simulink model "OORT"  (Simulink 7.6)
settings: Solver=ode3  SolverMode=SingleTasking  StartTime=0.0  StopTime=1.2  FixedStep=2e-5  RelTol=1e-4  AbsTol=1e-6
undefined symbols (not defined in the file or in its folder): DAB, den, elements, num
libraries: powerlib x179, powerlib_extras x6
(part 2 of 4)

== system OORT/Off-Line Analysis/Line 3 ==
  Fault : Subsystem
  Fault Selector : Subsystem
  Line1 : powerlib/Elements/Distributed Parameters Line  DialogController=POWERSYS.PowerSysDialog  SystemSampleTime=-1  Phases=3  Frequency=ff  Resistance=rr  Inductance=ll  Capacitance=cc  Length=length*faultLocation  x1=[0 5.77041232459445e-009 110738.683831382 -249234.318095428;3.63428122191995e-005 5.73023176322571e-009 114142.922310078 -247693.751838263;7.26856244383991e-005 5.68897556743528e-009 117525.734769496 -246106.690441544;0.000109028436657599 5.64665148151452e-009 120886.486214459 -244473.431816059;0.000145371248876798 5.6032674502108e-009 124224.545790915 -242794.282544381;0.000181714061095998 5.55883161723614e-009 127539.286904351 -241069.557823317]  x2=[0 6.14623169531121e-009 110795.572141665 -250854.024226143;3.63428122191995e-005 6.10087361816961e-009 114221.996046724 -249312.526552019;7.26856244383991e-005 6.05437033260761e-009 117626.979089399 -247724.229874574;0.000109028436657599 6.00673056785934e-009 121009.882112826 -246089.432336475;0.000145371248876798 5.95796326648995e-009 124370.07010483 -244408.440809168;0.000181714061095998 5.90807758271694e-009 127706.912317124 -242681.570835272]  x3=[0 1.63289630452373e-011 297.327539148724 -989.32395322872;3.63428122191995e-005 1.63493812805236e-011 310.853854870665 -985.157566524455;7.26856244383991e-005 1.63667305374499e-011 324.321819531038 -980.806253724158;0.000109028436657599 1.63810075593491e-011 337.728905028542 -976.270831622334;0.000145371248876798 1.639220966625e-011 351.072594689637 -971.552151573052;0.000181714061095998 1.64003347553804e-011 364.350383740955 -966.651099330137]  x4=[0 -1.69443168699963e-012 498.560173361075 -967.719754733797;3.63428122191995e-005 -1.84264732192147e-012 511.771614093406 -960.798410267261;7.26856244383991e-005 -1.99051706945717e-012 524.886989049184 -953.696712215548;0.000109028436657599 -2.13801317265084e-012 537.903836312498 -946.415993654038;0.000145371248876798 -2.28510794468418e-012 550.819712462286 -938.957621262444;0.000181714061095998 -2.43177377407364e-012 563.632193030996 -931.32299506827]  x5=0.000181714061095998  Measurements=None
  Line2 : powerlib/Elements/Distributed Parameters Line  DialogController=POWERSYS.PowerSysDialog  SystemSampleTime=-1  Phases=3  Frequency=ff  Resistance=rr  Inductance=ll  Capacitance=cc  Length=length*(1-faultLocation)  x1=[0 6.14623169531121e-009 110795.572141665 -250854.024226143;3.63428122191995e-005 6.10087361816961e-009 114221.996046724 -249312.526552019;7.26856244383991e-005 6.05437033260761e-009 117626.979089399 -247724.229874574;0.000109028436657599 6.00673056785934e-009 121009.882112826 -246089.432336475;0.000145371248876798 5.95796326648995e-009 124370.07010483 -244408.440809168;0.000181714061095998 5.90807758271694e-009 127706.912317124 -242681.570835272]  x2=[0 6.09065079529943e-009 110951.105544523 -251348.844420414;3.63428122191995e-005 6.04474609507565e-009 114384.294130345 -249805.169420755;7.26856244383991e-005 5.99770672225242e-009 117796.011388453 -248214.602942697;0.000109028436657599 5.94954150669399e-009 121185.616897888 -246577.443554977;0.000145371248876798 5.90025948959903e-009 124552.474388336 -244893.998572387;0.000181714061095998 5.84986992180347e-009 127895.951859564 -243164.583998093]  x3=[0 1.03895542727053e-011 368.109218234945 -994.520254979836;3.63428122191995e-005 1.03400987350235e-011 381.70008253833 -989.383636970479;7.26856244383991e-005 1.02887022346403e-011 395.219297078756 -984.0612995801;0.000109028436657599 1.02353744193059e-011 408.664324134692 -978.554241876369;0.000145371248876798 1.01801252993019e-011 422.032639910506 -972.863497601215;0.000181714061095998 1.01229652455624e-011 435.321735010208 -966.990134976776]  x4=[0 6.77730234632808e-012 428.347420618646 -970.712392687894;3.63428122191995e-005 6.74770065951855e-012 441.606451848913 -964.752716375506;7.26856244383991e-005 6.71683234696046e-012 454.782588159728 -958.611944206436;0.000109028436657599 6.6847032030127e-012 467.873356229534 -952.291228878548;0.000145371248876798 6.65131925870764e-012 480.87629876143 -945.791756867236;0.000181714061095998 6.61668678061897e-012 493.788974944442 -939.1147482027]  x5=0.000181714061095998  Measurements=None
  Timer : powerlib_extras/Control  Blocks/Timer  DialogController=POWERSYS.PowerSysDialog  SystemSampleTime=-1  t=[0 faultTime]  e=[0 1 0 1 0 1]
  A1 : PMIOPort  Tag=PMCPort  Port=1  Side=Left
  B1 : PMIOPort  Tag=PMCPort  Port=2  Side=Left
  C1 : PMIOPort  Tag=PMCPort  Port=3  Side=Left
  A2 : PMIOPort  Tag=PMCPort  Port=4  Side=Right
  B2 : PMIOPort  Tag=PMCPort  Port=5  Side=Right
  C2 : PMIOPort  Tag=PMCPort  Port=6  Side=Right
  wires:
  Fault Selector/1(faultA) -> Fault/1(faultA)
  Fault Selector/2(faultB) -> Fault/2(faultB)
  Fault Selector/3(faultC) -> Fault/3(faultC)
  Fault Selector/4(faultG) -> Fault/4(faultG)
  Timer/1 -> Fault/5(Tfault)
  connections:
  Line1/RConn1 -- Line2/LConn1 -- Fault/LConn1
  Line1/RConn2 -- Line2/LConn2 -- Fault/LConn2
  Line2/LConn3 -- Line1/RConn3 -- Fault/LConn3
  A1/RConn1 -- Line1/LConn1
  B1/RConn1 -- Line1/LConn2
  C1/RConn1 -- Line1/LConn3
  Line2/RConn1 -- A2/RConn1
  Line2/RConn2 -- B2/RConn1
  Line2/RConn3 -- C2/RConn1

== system OORT/On-Line Analysis/CB-1 ==
  Trip : Inport
  BreakerA : powerlib/Elements/Breaker  DialogController=POWERSYS.PowerSysDialog  SystemSampleTime=-1  BreakerResistance=0.01  InitialState=1  SnubberResistance=1e6  SnubberCapacitance=inf  SwitchingTimes="[ 1/60  5/60 ]"  External=on  Measurements=None  MoreParameters=off  NoBreakLoop=off
  BreakerB : powerlib/Elements/Breaker  DialogController=POWERSYS.PowerSysDialog  SystemSampleTime=-1  BreakerResistance=0.01  InitialState=1  SnubberResistance=1e6  SnubberCapacitance=inf  SwitchingTimes="[ 1/60  5/60 ]"  External=on  Measurements=None  MoreParameters=off  NoBreakLoop=off
  BreakerC : powerlib/Elements/Breaker  DialogController=POWERSYS.PowerSysDialog  SystemSampleTime=-1  BreakerResistance=0.01  InitialState=1  SnubberResistance=1e6  SnubberCapacitance=inf  SwitchingTimes="[ 1/60  5/60 ]"  External=on  Measurements=None  MoreParameters=off  NoBreakLoop=off
  NOT : Logic  Operator=NOT  Inputs=1
  Series RLC Branch1 : powerlib/Elements/Series RLC Branch  DialogController=POWERSYS.PowerSysDialog  PhysicalDomain=powersysdomain  SubClassName=unknown  LeftPortType=p1  RightPortType=p1  LConnTagsString=__new0  RConnTagsString=__new0  BranchType=R  Resistance=1e6  Inductance=1.0  SetiL0=off  InitialCurrent=0  Capacitance=1.0  Setx0=off  InitialVoltage=0  Measurements=None
  Series RLC Branch2 : powerlib/Elements/Series RLC Branch  DialogController=POWERSYS.PowerSysDialog  PhysicalDomain=powersysdomain  SubClassName=unknown  LeftPortType=p1  RightPortType=p1  LConnTagsString=__new0  RConnTagsString=__new0  BranchType=R  Resistance=1e6  Inductance=1.0  SetiL0=off  InitialCurrent=0  Capacitance=1.0  Setx0=off  InitialVoltage=0  Measurements=None
  Series RLC Branch3 : powerlib/Elements/Series RLC Branch  DialogController=POWERSYS.PowerSysDialog  PhysicalDomain=powersysdomain  SubClassName=unknown  LeftPortType=p1  RightPortType=p1  LConnTagsString=__new0  RConnTagsString=__new0  BranchType=R  Resistance=1e6  Inductance=1.0  SetiL0=off  InitialCurrent=0  Capacitance=1.0  Setx0=off  InitialVoltage=0  Measurements=None
  Transport Delay : TransportDelay  DelayTime=t_op+0.001  BufferSize=10240
  A1 : PMIOPort  Tag=PMCPort  Port=1  Side=Left
  B1 : PMIOPort  Tag=PMCPort  Port=2  Side=Left
  C1 : PMIOPort  Tag=PMCPort  Port=3  Side=Left
  A2 : PMIOPort  Tag=PMCPort  Port=4  Side=Right
  B2 : PMIOPort  Tag=PMCPort  Port=5  Side=Right
  C2 : PMIOPort  Tag=PMCPort  Port=6  Side=Right
  wires:
  NOT/1 -> BreakerA/1, BreakerB/1, BreakerC/1
  Transport Delay/1 -> NOT/1
  Trip/1 -> Transport Delay/1
  connections:
  A2/RConn1 -- BreakerA/RConn1 -- Series RLC Branch1/RConn1
  B2/RConn1 -- BreakerB/RConn1 -- Series RLC Branch2/RConn1
  C2/RConn1 -- BreakerC/RConn1 -- Series RLC Branch3/RConn1
  A1/RConn1 -- BreakerA/LConn1 -- Series RLC Branch1/LConn1
  B1/RConn1 -- BreakerB/LConn1 -- Series RLC Branch2/LConn1
  C1/RConn1 -- BreakerC/LConn1 -- Series RLC Branch3/LConn1

== system OORT/On-Line Analysis/CB-2 ==
  Trip : Inport
  BreakerA : powerlib/Elements/Breaker  DialogController=POWERSYS.PowerSysDialog  SystemSampleTime=-1  BreakerResistance=0.01  InitialState=1  SnubberResistance=1e6  SnubberCapacitance=inf  SwitchingTimes="[ 1/60  5/60 ]"  External=on  Measurements=None  MoreParameters=off  NoBreakLoop=off
  BreakerB : powerlib/Elements/Breaker  DialogController=POWERSYS.PowerSysDialog  SystemSampleTime=-1  BreakerResistance=0.01  InitialState=1  SnubberResistance=1e6  SnubberCapacitance=inf  SwitchingTimes="[ 1/60  5/60 ]"  External=on  Measurements=None  MoreParameters=off  NoBreakLoop=off
  BreakerC : powerlib/Elements/Breaker  DialogController=POWERSYS.PowerSysDialog  SystemSampleTime=-1  BreakerResistance=0.01  InitialState=1  SnubberResistance=1e6  SnubberCapacitance=inf  SwitchingTimes="[ 1/60  5/60 ]"  External=on  Measurements=None  MoreParameters=off  NoBreakLoop=off
  NOT : Logic  Operator=NOT  Inputs=1
  Series RLC Branch1 : powerlib/Elements/Series RLC Branch  DialogController=POWERSYS.PowerSysDialog  PhysicalDomain=powersysdomain  SubClassName=unknown  LeftPortType=p1  RightPortType=p1  LConnTagsString=__new0  RConnTagsString=__new0  BranchType=R  Resistance=1e6  Inductance=1.0  SetiL0=off  InitialCurrent=0  Capacitance=1.0  Setx0=off  InitialVoltage=0  Measurements=None
  Series RLC Branch2 : powerlib/Elements/Series RLC Branch  DialogController=POWERSYS.PowerSysDialog  PhysicalDomain=powersysdomain  SubClassName=unknown  LeftPortType=p1  RightPortType=p1  LConnTagsString=__new0  RConnTagsString=__new0  BranchType=R  Resistance=1e6  Inductance=1.0  SetiL0=off  InitialCurrent=0  Capacitance=1.0  Setx0=off  InitialVoltage=0  Measurements=None
  Series RLC Branch3 : powerlib/Elements/Series RLC Branch  DialogController=POWERSYS.PowerSysDialog  PhysicalDomain=powersysdomain  SubClassName=unknown  LeftPortType=p1  RightPortType=p1  LConnTagsString=__new0  RConnTagsString=__new0  BranchType=R  Resistance=1e6  Inductance=1.0  SetiL0=off  InitialCurrent=0  Capacitance=1.0  Setx0=off  InitialVoltage=0  Measurements=None
  Transport Delay : TransportDelay  DelayTime=t_op+0.001  BufferSize=10240
  A1 : PMIOPort  Tag=PMCPort  Port=1  Side=Left
  B1 : PMIOPort  Tag=PMCPort  Port=2  Side=Left
  C1 : PMIOPort  Tag=PMCPort  Port=3  Side=Left
  A2 : PMIOPort  Tag=PMCPort  Port=4  Side=Right
  B2 : PMIOPort  Tag=PMCPort  Port=5  Side=Right
  C2 : PMIOPort  Tag=PMCPort  Port=6  Side=Right
  wires:
  Trip/1 -> Transport Delay/1
  Transport Delay/1 -> NOT/1
  NOT/1 -> BreakerC/1, BreakerB/1, BreakerA/1
  connections:
  Series RLC Branch3/LConn1 -- BreakerC/LConn1 -- C1/RConn1
  Series RLC Branch2/LConn1 -- BreakerB/LConn1 -- B1/RConn1
  Series RLC Branch1/LConn1 -- BreakerA/LConn1 -- A1/RConn1
  Series RLC Branch3/RConn1 -- BreakerC/RConn1 -- C2/RConn1
  Series RLC Branch2/RConn1 -- BreakerB/RConn1 -- B2/RConn1
  Series RLC Branch1/RConn1 -- BreakerA/RConn1 -- A2/RConn1

== system OORT/On-Line Analysis/CB-3 ==
  Trip : Inport
  BreakerA : powerlib/Elements/Breaker  DialogController=POWERSYS.PowerSysDialog  SystemSampleTime=-1  BreakerResistance=0.01  InitialState=1  SnubberResistance=1e6  SnubberCapacitance=inf  SwitchingTimes="[ 1/60  5/60 ]"  External=on  Measurements=None  MoreParameters=off  NoBreakLoop=off
  BreakerB : powerlib/Elements/Breaker  DialogController=POWERSYS.PowerSysDialog  SystemSampleTime=-1  BreakerResistance=0.01  InitialState=1  SnubberResistance=1e6  SnubberCapacitance=inf  SwitchingTimes="[ 1/60  5/60 ]"  External=on  Measurements=None  MoreParameters=off  NoBreakLoop=off
  BreakerC : powerlib/Elements/Breaker  DialogController=POWERSYS.PowerSysDialog  SystemSampleTime=-1  BreakerResistance=0.01  InitialState=1  SnubberResistance=1e6  SnubberCapacitance=inf  SwitchingTimes="[ 1/60  5/60 ]"  External=on  Measurements=None  MoreParameters=off  NoBreakLoop=off
  NOT : Logic  Operator=NOT  Inputs=1
  Series RLC Branch1 : powerlib/Elements/Series RLC Branch  DialogController=POWERSYS.PowerSysDialog  PhysicalDomain=powersysdomain  SubClassName=unknown  LeftPortType=p1  RightPortType=p1  LConnTagsString=__new0  RConnTagsString=__new0  BranchType=R  Resistance=1e6  Inductance=1.0  SetiL0=off  InitialCurrent=0  Capacitance=1.0  Setx0=off  InitialVoltage=0  Measurements=None
  Series RLC Branch2 : powerlib/Elements/Series RLC Branch  DialogController=POWERSYS.PowerSysDialog  PhysicalDomain=powersysdomain  SubClassName=unknown  LeftPortType=p1  RightPortType=p1  LConnTagsString=__new0  RConnTagsString=__new0  BranchType=R  Resistance=1e6  Inductance=1.0  SetiL0=off  InitialCurrent=0  Capacitance=1.0  Setx0=off  InitialVoltage=0  Measurements=None
  Series RLC Branch3 : powerlib/Elements/Series RLC Branch  DialogController=POWERSYS.PowerSysDialog  PhysicalDomain=powersysdomain  SubClassName=unknown  LeftPortType=p1  RightPortType=p1  LConnTagsString=__new0  RConnTagsString=__new0  BranchType=R  Resistance=1e6  Inductance=1.0  SetiL0=off  InitialCurrent=0  Capacitance=1.0  Setx0=off  InitialVoltage=0  Measurements=None
  Transport Delay : TransportDelay  DelayTime=t_op+0.001  BufferSize=10240
  A1 : PMIOPort  Tag=PMCPort  Port=1  Side=Left
  B1 : PMIOPort  Tag=PMCPort  Port=2  Side=Left
  C1 : PMIOPort  Tag=PMCPort  Port=3  Side=Left
  A2 : PMIOPort  Tag=PMCPort  Port=4  Side=Right
  B2 : PMIOPort  Tag=PMCPort  Port=5  Side=Right
  C2 : PMIOPort  Tag=PMCPort  Port=6  Side=Right
  wires:
  NOT/1 -> BreakerA/1, BreakerB/1, BreakerC/1
  Transport Delay/1 -> NOT/1
  Trip/1 -> Transport Delay/1
  connections:
  A2/RConn1 -- BreakerA/RConn1 -- Series RLC Branch1/RConn1
  B2/RConn1 -- BreakerB/RConn1 -- Series RLC Branch2/RConn1
  C2/RConn1 -- BreakerC/RConn1 -- Series RLC Branch3/RConn1
  A1/RConn1 -- BreakerA/LConn1 -- Series RLC Branch1/LConn1
  B1/RConn1 -- BreakerB/LConn1 -- Series RLC Branch2/LConn1
  C1/RConn1 -- BreakerC/LConn1 -- Series RLC Branch3/LConn1

== system OORT/On-Line Analysis/CT-1 ==
  CT-ratio : Gain  Gain=1/CT  SaturateOnIntegerOverflow=on  OutDataTypeStr=Inherit: Same as input  ParamDataTypeStr=Inherit: Same as input
  Ground : powerlib/Elements/Ground  DialogController=POWERSYS.PowerSysDialog  PhysicalDomain=powersysdomain  SubClassName=unknown  LeftPortType=p1  RightPortType=p1  LConnTagsString=a
  IA : powerlib/Measurements/Current Measurement  DialogController=POWERSYS.PowerSysDialog  SystemSampleTime=-1  PhasorSimulation=off  OutputType=Complex  PSBequivalent=0
  IB : powerlib/Measurements/Current Measurement  DialogController=POWERSYS.PowerSysDialog  SystemSampleTime=-1  PhasorSimulation=off  OutputType=Complex  PSBequivalent=0
  IC : powerlib/Measurements/Current Measurement  DialogController=POWERSYS.PowerSysDialog  SystemSampleTime=-1  PhasorSimulation=off  OutputType=Complex  PSBequivalent=0
  Mux : Mux  Inputs=3
  Mux1 : Mux  Inputs=3
  VA : powerlib/Measurements/Voltage Measurement  DialogController=POWERSYS.PowerSysDialog  SystemSampleTime=-1  PhasorSimulation=off  OutputType=Complex  PSBequivalent=0
  VB : powerlib/Measurements/Voltage Measurement  DialogController=POWERSYS.PowerSysDialog  SystemSampleTime=-1  PhasorSimulation=off  OutputType=Complex  PSBequivalent=0
  VC : powerlib/Measurements/Voltage Measurement  DialogController=POWERSYS.PowerSysDialog  SystemSampleTime=-1  PhasorSimulation=off  OutputType=Complex  PSBequivalent=0
  VT-ratio : Gain  Gain=1/VT  SaturateOnIntegerOverflow=on  OutDataTypeStr=Inherit: Same as input  ParamDataTypeStr=Inherit: Same as input
  A1 : PMIOPort  Tag=PMCPort  Port=1  Side=Left
  B1 : PMIOPort  Tag=PMCPort  Port=2  Side=Left
  C1 : PMIOPort  Tag=PMCPort  Port=3  Side=Left
  A2 : PMIOPort  Tag=PMCPort  Port=4  Side=Right
  B2 : PMIOPort  Tag=PMCPort  Port=5  Side=Right
  C2 : PMIOPort  Tag=PMCPort  Port=6  Side=Right
  Vabc : Outport  InitialOutput=0
  Iabc : Outport  Port=2  InitialOutput=0
  wires:
  VC/1 -> Mux1/3
  VB/1 -> Mux1/2
  VA/1 -> Mux1/1
  CT-ratio/1 -> Iabc/1
  Mux/1 -> CT-ratio/1
  VT-ratio/1 -> Vabc/1
  Mux1/1 -> VT-ratio/1
  IA/1 -> Mux/1
  IB/1 -> Mux/2
  IC/1 -> Mux/3
  connections:
  IC/RConn1 -- C2/RConn1
  IB/RConn1 -- B2/RConn1
  A2/RConn1 -- IA/RConn1
  VC/LConn1 -- IC/LConn1 -- C1/RConn1
  VB/LConn1 -- IB/LConn1 -- B1/RConn1
  VA/LConn1 -- IA/LConn1 -- A1/RConn1
  VC/LConn2 -- Ground/LConn1 -- VB/LConn2 -- VA/LConn2

== system OORT/On-Line Analysis/CT-2 ==
  CT-ratio : Gain  Gain=1/CT  SaturateOnIntegerOverflow=on  OutDataTypeStr=Inherit: Same as input  ParamDataTypeStr=Inherit: Same as input
  Ground : powerlib/Elements/Ground  DialogController=POWERSYS.PowerSysDialog  PhysicalDomain=powersysdomain  SubClassName=unknown  LeftPortType=p1  RightPortType=p1  LConnTagsString=a
  IA : powerlib/Measurements/Current Measurement  DialogController=POWERSYS.PowerSysDialog  SystemSampleTime=-1  PhasorSimulation=off  OutputType=Complex  PSBequivalent=0
  IB : powerlib/Measurements/Current Measurement  DialogController=POWERSYS.PowerSysDialog  SystemSampleTime=-1  PhasorSimulation=off  OutputType=Complex  PSBequivalent=0
  IC : powerlib/Measurements/Current Measurement  DialogController=POWERSYS.PowerSysDialog  SystemSampleTime=-1  PhasorSimulation=off  OutputType=Complex  PSBequivalent=0
  Mux : Mux  Inputs=3
  Mux1 : Mux  Inputs=3
  VA : powerlib/Measurements/Voltage Measurement  DialogController=POWERSYS.PowerSysDialog  SystemSampleTime=-1  PhasorSimulation=off  OutputType=Complex  PSBequivalent=0
  VB : powerlib/Measurements/Voltage Measurement  DialogController=POWERSYS.PowerSysDialog  SystemSampleTime=-1  PhasorSimulation=off  OutputType=Complex  PSBequivalent=0
  VC : powerlib/Measurements/Voltage Measurement  DialogController=POWERSYS.PowerSysDialog  SystemSampleTime=-1  PhasorSimulation=off  OutputType=Complex  PSBequivalent=0
  VT-ratio : Gain  Gain=1/VT  SaturateOnIntegerOverflow=on  OutDataTypeStr=Inherit: Same as input  ParamDataTypeStr=Inherit: Same as input
  A1 : PMIOPort  Tag=PMCPort  Port=1  Side=Left
  B1 : PMIOPort  Tag=PMCPort  Port=2  Side=Left
  C1 : PMIOPort  Tag=PMCPort  Port=3  Side=Left
  A2 : PMIOPort  Tag=PMCPort  Port=4  Side=Right
  B2 : PMIOPort  Tag=PMCPort  Port=5  Side=Right
  C2 : PMIOPort  Tag=PMCPort  Port=6  Side=Right
  Vabc : Outport  InitialOutput=0
  Iabc : Outport  Port=2  InitialOutput=0
  wires:
  IC/1 -> Mux/3
  IB/1 -> Mux/2
  IA/1 -> Mux/1
  Mux1/1 -> VT-ratio/1
  VT-ratio/1 -> Vabc/1
  Mux/1 -> CT-ratio/1
  CT-ratio/1 -> Iabc/1
  VA/1 -> Mux1/1
  VB/1 -> Mux1/2
  VC/1 -> Mux1/3
  connections:
  VA/LConn2 -- VB/LConn2 -- Ground/LConn1 -- VC/LConn2
  A1/RConn1 -- IA/LConn1 -- VA/LConn1
  B1/RConn1 -- IB/LConn1 -- VB/LConn1
  C1/RConn1 -- IC/LConn1 -- VC/LConn1
  A2/RConn1 -- IA/RConn1
  IB/RConn1 -- B2/RConn1
  IC/RConn1 -- C2/RConn1

== system OORT/On-Line Analysis/CT-3 ==
  CT-ratio : Gain  Gain=1/CT  SaturateOnIntegerOverflow=on  OutDataTypeStr=Inherit: Same as input  ParamDataTypeStr=Inherit: Same as input
  Ground : powerlib/Elements/Ground  DialogController=POWERSYS.PowerSysDialog  PhysicalDomain=powersysdomain  SubClassName=unknown  LeftPortType=p1  RightPortType=p1  LConnTagsString=a
  IA : powerlib/Measurements/Current Measurement  DialogController=POWERSYS.PowerSysDialog  SystemSampleTime=-1  PhasorSimulation=off  OutputType=Complex  PSBequivalent=0
  IB : powerlib/Measurements/Current Measurement  DialogController=POWERSYS.PowerSysDialog  SystemSampleTime=-1  PhasorSimulation=off  OutputType=Complex  PSBequivalent=0
  IC : powerlib/Measurements/Current Measurement  DialogController=POWERSYS.PowerSysDialog  SystemSampleTime=-1  PhasorSimulation=off  OutputType=Complex  PSBequivalent=0
  Mux : Mux  Inputs=3
  Mux1 : Mux  Inputs=3
  VA : powerlib/Measurements/Voltage Measurement  DialogController=POWERSYS.PowerSysDialog  SystemSampleTime=-1  PhasorSimulation=off  OutputType=Complex  PSBequivalent=0
  VB : powerlib/Measurements/Voltage Measurement  DialogController=POWERSYS.PowerSysDialog  SystemSampleTime=-1  PhasorSimulation=off  OutputType=Complex  PSBequivalent=0
  VC : powerlib/Measurements/Voltage Measurement  DialogController=POWERSYS.PowerSysDialog  SystemSampleTime=-1  PhasorSimulation=off  OutputType=Complex  PSBequivalent=0
  VT-ratio : Gain  Gain=1/VT  SaturateOnIntegerOverflow=on  OutDataTypeStr=Inherit: Same as input  ParamDataTypeStr=Inherit: Same as input
  A1 : PMIOPort  Tag=PMCPort  Port=1  Side=Left
  B1 : PMIOPort  Tag=PMCPort  Port=2  Side=Left
  C1 : PMIOPort  Tag=PMCPort  Port=3  Side=Left
  A2 : PMIOPort  Tag=PMCPort  Port=4  Side=Right
  B2 : PMIOPort  Tag=PMCPort  Port=5  Side=Right
  C2 : PMIOPort  Tag=PMCPort  Port=6  Side=Right
  Vabc : Outport  InitialOutput=0
  Iabc : Outport  Port=2  InitialOutput=0
  wires:
  IC/1 -> Mux/3
  IB/1 -> Mux/2
  IA/1 -> Mux/1
  Mux1/1 -> VT-ratio/1
  VT-ratio/1 -> Vabc/1
  Mux/1 -> CT-ratio/1
  CT-ratio/1 -> Iabc/1
  VA/1 -> Mux1/1
  VB/1 -> Mux1/2
  VC/1 -> Mux1/3
  connections:
  VA/LConn2 -- VB/LConn2 -- Ground/LConn1 -- VC/LConn2
  A1/RConn1 -- IA/LConn1 -- VA/LConn1
  B1/RConn1 -- IB/LConn1 -- VB/LConn1
  C1/RConn1 -- IC/LConn1 -- VC/LConn1
  A2/RConn1 -- IA/RConn1
  IB/RConn1 -- B2/RConn1
  IC/RConn1 -- C2/RConn1

== system OORT/On-Line Analysis/Generator ==
  Ground : powerlib/Elements/Ground  DialogController=POWERSYS.PowerSysDialog  PhysicalDomain=powersysdomain  SubClassName=unknown  LeftPortType=p1  RightPortType=p1  LConnTagsString=a
  RA : powerlib/Elements/Series RLC Branch  DialogController=POWERSYS.PowerSysDialog  PhysicalDomain=powersysdomain  SubClassName=unknown  LeftPortType=p1  RightPortType=p1  LConnTagsString=__new0  RConnTagsString=__new0  BranchType=RL  Resistance=R  Inductance=L  SetiL0=off  InitialCurrent=0  Capacitance=1.0  Setx0=off  InitialVoltage=0  Measurements=None
  RB : powerlib/Elements/Series RLC Branch  DialogController=POWERSYS.PowerSysDialog  PhysicalDomain=powersysdomain  SubClassName=unknown  LeftPortType=p1  RightPortType=p1  LConnTagsString=__new0  RConnTagsString=__new0  BranchType=RL  Resistance=R  Inductance=L  SetiL0=off  InitialCurrent=0  Capacitance=1.0  Setx0=off  InitialVoltage=0  Measurements=None
  RC : powerlib/Elements/Series RLC Branch  DialogController=POWERSYS.PowerSysDialog  PhysicalDomain=powersysdomain  SubClassName=unknown  LeftPortType=p1  RightPortType=p1  LConnTagsString=__new0  RConnTagsString=__new0  BranchType=RL  Resistance=R  Inductance=L  SetiL0=off  InitialCurrent=0  Capacitance=1.0  Setx0=off  InitialVoltage=0  Measurements=None
  VA : powerlib/Electrical Sources/AC Voltage Source  DialogController=POWERSYS.PowerSysDialog  SystemSampleTime=-1  Amplitude=V  Phase=Phi  Frequency=F  SampleTime=0  Measurements=None
  VB : powerlib/Electrical Sources/AC Voltage Source  DialogController=POWERSYS.PowerSysDialog  SystemSampleTime=-1  Amplitude=V  Phase=Phi-120  Frequency=F  SampleTime=0  Measurements=None
  VC : powerlib/Electrical Sources/AC Voltage Source  DialogController=POWERSYS.PowerSysDialog  SystemSampleTime=-1  Amplitude=V  Phase=Phi+120  Frequency=F  SampleTime=0  Measurements=None
  A : PMIOPort  Tag=PMCPort  Port=1  Side=Right
  B : PMIOPort  Tag=PMCPort  Port=2  Side=Right
  C : PMIOPort  Tag=PMCPort  Port=3  Side=Right
  connections:
  VC/LConn1 -- VA/LConn1 -- Ground/LConn1 -- VB/LConn1
  VA/RConn1 -- RA/LConn1
  VB/RConn1 -- RB/LConn1
  VC/RConn1 -- RC/LConn1
  RA/RConn1 -- A/RConn1
  RB/RConn1 -- B/RConn1
  RC/RConn1 -- C/RConn1

== system OORT/On-Line Analysis/Line 1 ==
  Fault : Subsystem
  Fault Selector : Subsystem
  Line1 : powerlib/Elements/Distributed Parameters Line  DialogController=POWERSYS.PowerSysDialog  SystemSampleTime=-1  Phases=3  Frequency=ff  Resistance=rr  Inductance=ll  Capacitance=cc  Length=length*faultLocation  x1=[0 -7.01834070085229e-010 108952.627247472 -232501.161061733;3.63428122191995e-005 -7.01428749440589e-010 112127.780928205 -230986.635161641;7.26856244383991e-005 -7.00891762060913e-010 115281.886856286 -229428.750251652;0.000109028436657599 -7.00223208745285e-010 118414.352967545 -227827.798765774;0.000145371248876798 -6.99423214989321e-010 121524.591259872 -226184.081222135;0.000181714061095998 -6.98491930961609e-010 124612.017903589 -224497.906166575]  x2=[0 -1.52877524817155e-009 109483.947277545 -238248.017098747;3.63428122191995e-005 -1.52627193399432e-009 112737.785827333 -236725.672477041;7.26856244383991e-005 -1.52348211995166e-009 115970.462119106 -235158.891558108;0.000109028436657599 -1.52040632972569e-009 119181.369340079 -233547.968445843;0.000145371248876798 -1.51704514067979e-009 122369.904763788 -231893.205530172;0.000181714061095998 -1.51339918375015e-009 125535.469863226 -230194.913430284]  x3=[0 -6.71379139484889e-012 38.1880834031549 -980.547626715663;3.63428122191995e-005 -6.9572162636958e-012 51.6184809810537 -979.932400930255;7.26856244383991e-005 -7.19933517815874e-012 65.0391891402286 -979.133229876152;0.000109028436657599 -7.44010268956315e-012 78.4476886500001 -978.150263567514;0.000145371248876798 -7.67947360290931e-012 91.841462571401 -976.98368651911;0.000181714061095998 -7.91740298535603e-012 105.217996729637 -975.633717711686]  x4=[0 3.82078051627435e-012 749.225398635594 -862.856254941147;3.63428122191995e-005 4.04224476213212e-012 760.976631704422 -852.51051644629;7.26856244383991e-005 4.26295022932497e-012 772.585020174116 -842.004751325245;0.000109028436657599 4.48285548874366e-012 784.048385008516 -831.340931638317;0.000145371248876798 4.70191926148775e-012 795.364574394168 -820.521059114579;0.000181714061095998 4.92010042661411e-012 806.531464144245 -809.547164776127]  x5=0.000181714061095998  Measurements=None
  Line2 : powerlib/Elements/Distributed Parameters Line  DialogController=POWERSYS.PowerSysDialog  SystemSampleTime=-1  Phases=3  Frequency=ff  Resistance=rr  Inductance=ll  Capacitance=cc  Length=length*(1-faultLocation)  x1=[0 -1.52877524817155e-009 109483.947277545 -238248.017098747;3.63428122191995e-005 -1.52627193399432e-009 112737.785827333 -236725.672477041;7.26856244383991e-005 -1.52348211995166e-009 115970.462119106 -235158.891558108;0.000109028436657599 -1.52040632972569e-009 119181.369340079 -233547.968445843;0.000145371248876798 -1.51704514067979e-009 122369.904763788 -231893.205530172;0.000181714061095998 -1.51339918375015e-009 125535.469863226 -230194.913430284]  x2=[0 -2.45883505016193e-009 110093.603783289 -242918.061375908;3.63428122191995e-005 -2.45402124181503e-009 113411.367002337 -241386.925849936;7.26856244383991e-005 -2.44874678373732e-009 116707.841523964 -239810.479052602;0.000109028436657599 -2.44301266600893e-009 119982.40855968 -238189.016902206;0.000145371248876798 -2.43681996499373e-009 123234.453433295 -236522.843766978;0.000181714061095998 -2.43016984313726e-009 126463.365696306 -234812.272407946]  x3=[0 -7.55932174289328e-012 107.184150432297 -1000.77656031182;3.63428122191995e-005 -7.79229810148879e-012 120.88521858622 -999.214156075072;7.26856244383991e-005 -8.02381175064978e-012 134.563595109585 -997.464187148912;0.000109028436657599 -8.25381923243941e-012 148.216712404216 -995.526982023864;0.000145371248876798 -8.48227737164681e-012 161.842007613402 -993.402904336966;0.000181714061095998 -8.70914328389163e-012 175.43692310298 -991.092352803518]  x4=[0 3.75555028169632e-012 683.39695405214 -882.980145406505;3.63428122191995e-005 4.01268402084736e-012 695.43007265773 -873.534400028471;7.26856244383991e-005 4.26906453024532e-012 707.332650553113 -863.92468158477;0.000109028436657599 4.52464368414023e-012 719.102453479182 -854.15279393681;0.000145371248876798 4.77937350720637e-012 730.737272100315 -844.22057138714;0.000181714061095998 5.03320618354776e-012 742.23492241909 -834.129878335123]  x5=0.000181714061095998  Measurements=None
  Timer : powerlib_extras/Control  Blocks/Timer  DialogController=POWERSYS.PowerSysDialog  SystemSampleTime=-1  t=[0 faultTime]  e=[0 1 0 1 0 1]
  A1 : PMIOPort  Tag=PMCPort  Port=1  Side=Left
  B1 : PMIOPort  Tag=PMCPort  Port=2  Side=Left
  C1 : PMIOPort  Tag=PMCPort  Port=3  Side=Left
  A2 : PMIOPort  Tag=PMCPort  Port=4  Side=Right
  B2 : PMIOPort  Tag=PMCPort  Port=5  Side=Right
  C2 : PMIOPort  Tag=PMCPort  Port=6  Side=Right
  wires:
  Timer/1 -> Fault/5(Tfault)
  Fault Selector/4(faultG) -> Fault/4(faultG)
  Fault Selector/3(faultC) -> Fault/3(faultC)
  Fault Selector/2(faultB) -> Fault/2(faultB)
  Fault Selector/1(faultA) -> Fault/1(faultA)
  connections:
  Line2/RConn3 -- C2/RConn1
  Line2/RConn2 -- B2/RConn1
  Line2/RConn1 -- A2/RConn1
  C1/RConn1 -- Line1/LConn3
  B1/RConn1 -- Line1/LConn2
  A1/RConn1 -- Line1/LConn1
  Fault/LConn3 -- Line1/RConn3 -- Line2/LConn3
  Fault/LConn2 -- Line2/LConn2 -- Line1/RConn2
  Fault/LConn1 -- Line2/LConn1 -- Line1/RConn1

== system OORT/On-Line Analysis/Line 2 ==
  Fault : Subsystem
  Fault Selector : Subsystem
  Line1 : powerlib/Elements/Distributed Parameters Line  DialogController=POWERSYS.PowerSysDialog  SystemSampleTime=-1  Phases=3  Frequency=ff  Resistance=rr  Inductance=ll  Capacitance=cc  Length=length*faultLocation  x1=[0 -2.46478129684385e-009 116025.27415649 -240140.830933759;2.18056873315197e-005 -2.46110148616177e-009 117995.42141564 -239178.936049123;4.36113746630395e-005 -2.45725536145418e-009 119957.594890028 -238200.878152967;6.54170619945592e-005 -2.45324318263091e-009 121911.661981722 -237206.723339578;8.72227493260789e-005 -2.44906522082326e-009 123857.490640594 -236196.538791024;0.000109028436657599 -2.44472175836563e-009 125794.949373247 -235170.392772617]  x2=[0 -2.93203184901205e-009 116294.487996897 -242477.692278278;2.18056873315197e-005 -2.93100843084219e-009 118283.836229933 -241513.505373489;4.36113746630395e-005 -2.92978694371268e-009 120265.191187978 -240532.997693827;6.54170619945592e-005 -2.92836747016805e-009 122238.418976873 -239536.235499129;8.72227493260789e-005 -2.92675010613216e-009 124203.386251667 -238523.286147661;0.000109028436657599 -2.92493496090174e-009 126159.960225629 -237494.218091572]  x3=[0 4.78068567214762e-012 191.549000901434 -990.17039243633;2.18056873315197e-005 4.65252613864933e-012 199.682182734816 -988.562315538131;4.36113746630395e-005 4.52405220107008e-012 207.801870631512 -986.887434495898;6.54170619945592e-005 4.39527254130203e-012 215.90751588681 -985.145862493183;8.72227493260789e-005 4.26619586189719e-012 223.99857074496 -983.337717220317;0.000109028436657599 4.13683088547924e-012 232.074488436187 -981.46312086646]  x4=[0 -9.75414812953871e-012 672.653293383239 -893.22468781442;2.18056873315197e-005 -9.59533151025605e-012 679.973281327228 -887.664989002928;4.36113746630395e-005 -9.43586646659165e-012 687.24731866971 -882.045304393023;6.54170619945592e-005 -9.2757637747258e-012 694.474913852561 -876.36601374652;8.72227493260789e-005 -9.11503425392919e-012 701.655578456081 -870.627500853235;0.000109028436657599 -8.95368876583178e-012 708.788827232001 -864.830153505053]  x5=0.000109028436657599  Measurements=None
  Line2 : powerlib/Elements/Distributed Parameters Line  DialogController=POWERSYS.PowerSysDialog  SystemSampleTime=-1  Phases=3  Frequency=ff  Resistance=rr  Inductance=ll  Capacitance=cc  Length=length*(1-faultLocation)  x1=[0 -2.93378916936335e-009 104244.412461385 -247897.038428538;5.08799371068794e-005 -2.93417644929558e-009 108979.928183501 -245852.017368535;0.000101759874213759 -2.93348421522405e-009 113675.349057663 -243716.544796774;0.000152639811320638 -2.93171272182886e-009 118328.947589743 -241491.406375803;0.000203519748427517 -2.92886262086083e-009 122939.011672488 -239177.420757168;0.000254399685534397 -2.92493496090174e-009 127503.845215418 -236775.439280222]  x2=[0 -4.53080996650885e-009 104767.060486678 -251827.437542501;5.08799371068794e-005 -4.5156244877883e-009 109577.86554531 -249771.669019478;0.000101759874213759 -4.49877766389831e-009 114348.355768621 -247624.006904126;0.000152639811320638 -4.48027569296044e-009 119076.776043687 -245385.241343654;0.000203519748427517 -4.46012538204205e-009 123761.386735559 -243056.196003173;0.000254399685534397 -4.43833414465189e-009 128400.464327287 -240637.727762666]  x3=[0 -2.02073591708651e-011 188.011547242469 -1013.81175332517;5.08799371068794e-005 -2.06286095393604e-011 207.421980680539 -1010.01917556417;0.000101759874213759 -2.1042270428061e-011 226.756101416663 -1005.8550012537;0.000152639811320638 -2.14481896468277e-011 246.006796226927 -1001.32076243676;0.000203519748427517 -2.18462178537622e-011 265.166982580683 -996.418127306915;0.000254399685534397 -2.22362086101514e-011 284.229611246284 -991.148899594581]  x4=[0 8.92160989197731e-012 534.376337850191 -946.578568501694;5.08799371068794e-005 9.31160649418014e-012 552.433515924957 -936.15504446843;0.000101759874213759 9.69817725959989e-012 570.287447969059 -925.387099267025;0.000152639811320638 1.00811799648352e-011 587.931565335381 -914.278694536403;0.000203519748427517 1.04604736992113e-011 605.359376569812 -902.83391717409;0.000254399685534397 1.0835918916622e-011 622.564469799511 -891.056977832596]  x5=0.000254399685534397  Measurements=None
  Timer : powerlib_extras/Control  Blocks/Timer  DialogController=POWERSYS.PowerSysDialog  SystemSampleTime=-1  t=[0 faultTime]  e=[0 1 0 1 0 1]
  A1 : PMIOPort  Tag=PMCPort  Port=1  Side=Left
  B1 : PMIOPort  Tag=PMCPort  Port=2  Side=Left
  C1 : PMIOPort  Tag=PMCPort  Port=3  Side=Left
  A2 : PMIOPort  Tag=PMCPort  Port=4  Side=Right
  B2 : PMIOPort  Tag=PMCPort  Port=5  Side=Right
  C2 : PMIOPort  Tag=PMCPort  Port=6  Side=Right
  wires:
  Timer/1 -> Fault/5(Tfault)
  Fault Selector/4(faultG) -> Fault/4(faultG)
  Fault Selector/3(faultC) -> Fault/3(faultC)
  Fault Selector/2(faultB) -> Fault/2(faultB)
  Fault Selector/1(faultA) -> Fault/1(faultA)
  connections:
  Line2/RConn3 -- C2/RConn1
  Line2/RConn2 -- B2/RConn1
  Line2/RConn1 -- A2/RConn1
  C1/RConn1 -- Line1/LConn3
  B1/RConn1 -- Line1/LConn2
  A1/RConn1 -- Line1/LConn1
  Fault/LConn3 -- Line1/RConn3 -- Line2/LConn3
  Fault/LConn2 -- Line2/LConn2 -- Line1/RConn2
  Fault/LConn1 -- Line2/LConn1 -- Line1/RConn1

== system OORT/On-Line Analysis/Line 3 ==
  Fault : Subsystem
  Fault Selector : Subsystem
  Line1 : powerlib/Elements/Distributed Parameters Line  DialogController=POWERSYS.PowerSysDialog  SystemSampleTime=-1  Phases=3  Frequency=ff  Resistance=rr  Inductance=ll  Capacitance=cc  Length=length*faultLocation  x1=[0 -4.56136732002832e-009 98547.7874704362 -254325.331830909;6.54170619945592e-005 -4.54517478134994e-009 104789.267661978 -251817.890963066;0.000130834123989118 -4.52621802089006e-009 110967.018560353 -249157.302959489;0.000196251185983678 -4.50450856751009e-009 117077.283066126 -246345.185899937;0.000261668247978237 -4.48005962416631e-009 123116.345122811 -243383.250019021;0.000327085309972796 -4.45288605988026e-009 129080.531976842 -240273.2966661]  x2=[0 -6.25524299720162e-009 98309.8175499685 -256519.672112812;6.54170619945592e-005 -6.23702288103197e-009 104605.480673784 -254017.432119489;0.000130834123989118 -6.21500961821146e-009 110837.52627747 -251360.707303794;0.000196251185983678 -6.18921659646299e-009 117002.164241389 -248551.113396025;0.000261668247978237 -6.15965950223119e-009 123095.64544095 -245590.359096298;0.000327085309972796 -6.12635631114244e-009 129114.264026705 -242480.245035374]  x3=[0 -9.03571923669181e-012 247.99145458009 -998.765594632143;6.54170619945592e-005 -9.51611282791048e-012 272.544756762366 -992.346628012101;0.000130834123989118 -9.99071904072907e-012 296.932306429212 -985.32414969099;0.000196251185983678 -1.04592492356795e-011 321.139271896649 -977.702430502928;0.000261668247978237 -1.09214184685226e-011 345.150931305908 -969.48610572009;0.000327085309972796 -1.13769456635415e-011 368.95268157677 -960.680172233689]  x4=[0 -4.80422875643923e-012 400.118507423892 -1008.03000661099;6.54170619945592e-005 -4.34373100974009e-012 424.854002877892 -997.85689878354;0.000130834123989118 -3.88059155255727e-012 449.331116477463 -987.076928094458;0.000196251185983678 -3.41509205066533e-012 473.534962068866 -975.696650557802;0.000261668247978237 -2.94751560513835e-012 497.450819690735 -963.722987273985;0.000327085309972796 -2.47814658017735e-012 521.064144526262 -951.163220220585]  x5=0.000327085309972796  Measurements=None
  Line2 : powerlib/Elements/Distributed Parameters Line  DialogController=POWERSYS.PowerSysDialog  SystemSampleTime=-1  Phases=3  Frequency=ff  Resistance=rr  Inductance=ll  Capacitance=cc  Length=length*(1-faultLocation)  x1=[0 -6.14531941366124e-009 123003.886936897 -245636.329165675;7.26856244383991e-006 -6.14161896647918e-009 123676.512913545 -245298.354175316;1.45371248876798e-005 -6.13787240433183e-009 124348.210252624 -244958.53733753;2.18056873315197e-005 -6.13407975535063e-009 125018.973910628 -244616.881203866;2.90742497753596e-005 -6.13024104801306e-009 125688.798851061 -244273.388339685;3.63428122191995e-005 -6.12635631114244e-009 126357.680044473 -243928.061324136]  x2=[0 -6.24667483887919e-009 123010.272810931 -245655.732898324;7.26856244383991e-006 -6.24307751312814e-009 123682.951933325 -245317.740336672;1.45371248876798e-005 -6.23943331060006e-009 124354.702369803 -244977.905782031;2.18056873315197e-005 -6.23574225865783e-009 125025.519076459 -244636.231786083;2.90742497753596e-005 -6.23200438501608e-009 125695.397016399 -244292.72091432;3.63428122191995e-005 -6.22821971774101e-009 126364.331159775 -243947.37574603]  x3=[0 -9.35270248779189e-012 464.992241864358 -957.497846122209;7.26856244383991e-006 -9.37892863176301e-012 467.61421264533 -956.220088920328;1.45371248876798e-005 -9.40508435310279e-012 470.232672297834 -954.935151843489;2.18056873315197e-005 -9.43116945541836e-012 472.847601160904 -953.643044539774;2.90742497753596e-005 -9.45718374284709e-012 475.458979600081 -952.343776711099;3.63428122191995e-005 -9.48312702005808e-012 478.066788007567 -951.037358113149]  x4=[0 -1.80284037531772e-011 476.724848749044 -952.337256497933;7.26856244383991e-006 -1.80118173552792e-011 479.332634537519 -951.027369215066;1.45371248876798e-005 -1.79950957138345e-011 481.936821208576 -949.710341047302;2.18056873315197e-005 -1.7978238954399e-011 484.537389208414 -948.386181883679;2.90742497753596e-005 -1.79612472035436e-011 487.134319010408 -947.054901666781;3.63428122191995e-005 -1.79441205888524e-011 489.727591115248 -945.716510392658]  x5=3.63428122191995e-005  Measurements=None
  Timer : powerlib_extras/Control  Blocks/Timer  DialogController=POWERSYS.PowerSysDialog  SystemSampleTime=-1  t=[0 faultTime]  e=[0 1 0 1 0 1]
  A1 : PMIOPort  Tag=PMCPort  Port=1  Side=Left
  B1 : PMIOPort  Tag=PMCPort  Port=2  Side=Left
  C1 : PMIOPort  Tag=PMCPort  Port=3  Side=Left
  A2 : PMIOPort  Tag=PMCPort  Port=4  Side=Right
  B2 : PMIOPort  Tag=PMCPort  Port=5  Side=Right
  C2 : PMIOPort  Tag=PMCPort  Port=6  Side=Right
  wires:
  Fault Selector/1(faultA) -> Fault/1(faultA)
  Fault Selector/2(faultB) -> Fault/2(faultB)
  Fault Selector/3(faultC) -> Fault/3(faultC)
  Fault Selector/4(faultG) -> Fault/4(faultG)
  Timer/1 -> Fault/5(Tfault)
  connections:
  Line1/RConn1 -- Line2/LConn1 -- Fault/LConn1
  Line1/RConn2 -- Line2/LConn2 -- Fault/LConn2
  Line2/LConn3 -- Line1/RConn3 -- Fault/LConn3
  A1/RConn1 -- Line1/LConn1
  B1/RConn1 -- Line1/LConn2
  C1/RConn1 -- Line1/LConn3
  Line2/RConn1 -- A2/RConn1
  Line2/RConn2 -- B2/RConn1
  Line2/RConn3 -- C2/RConn1

== system OORT/On-Line Analysis/OR-1 ==
  Iabc : Inport
  Overcurrent Relay Scheme : Subsystem  mask{fCut=250, fSampling=60*32, WindowSize=10, VoltageRange=110/sqrt(3), CurrentRange=40, Td=Td, Top=Iop, ResCurr=ResCurr}
      mask prompts: fCut "fCut (Hz):"; fSampling "fSampling (Hz):"; WindowSize "Window Size (samples):"; VoltageRange "Voltage Range (V):"; CurrentRange "Current Range (A):"; Td "Time Delay (s):"; Top "Pickup Current (A):"; ResCurr "Residual Current (A):"
  Trip : Outport  InitialOutput=0
  Logic : Outport  Port=2  InitialOutput=0
  FaultType : Outport  Port=3  InitialOutput=0
  wires:
  Iabc/1 -> Overcurrent Relay Scheme/1(Iabc)
  Overcurrent Relay Scheme/1("TRIP ") -> Trip/1
  Overcurrent Relay Scheme/2(Logic) -> Logic/1
  Overcurrent Relay Scheme/3(FaultType) -> FaultType/1

== system OORT/On-Line Analysis/OR-2 ==
  Iabc : Inport
  Overcurrent Relay Scheme : Subsystem  mask{fCut=250, fSampling=60*32, WindowSize=10, VoltageRange=110/sqrt(3), CurrentRange=40, Td=Td, Top=Iop, ResCurr=ResCurr}
      mask prompts: fCut "fCut (Hz):"; fSampling "fSampling (Hz):"; WindowSize "Window Size (samples):"; VoltageRange "Voltage Range (V):"; CurrentRange "Current Range (A):"; Td "Time Delay (s):"; Top "Pickup Current (A):"; ResCurr "Residual Current (A):"
  Trip : Outport  InitialOutput=0
  Logic : Outport  Port=2  InitialOutput=0
  FaultType : Outport  Port=3  InitialOutput=0
  wires:
  Overcurrent Relay Scheme/3(FaultType) -> FaultType/1
  Overcurrent Relay Scheme/2(Logic) -> Logic/1
  Overcurrent Relay Scheme/1("TRIP ") -> Trip/1
  Iabc/1 -> Overcurrent Relay Scheme/1(Iabc)

== system OORT/On-Line Analysis/OR-3 ==
  Iabc : Inport
  Overcurrent Relay Scheme : Subsystem  mask{fCut=250, fSampling=60*32, WindowSize=10, VoltageRange=110/sqrt(3), CurrentRange=40, Td=Td, Top=Iop, ResCurr=ResCurr}
      mask prompts: fCut "fCut (Hz):"; fSampling "fSampling (Hz):"; WindowSize "Window Size (samples):"; VoltageRange "Voltage Range (V):"; CurrentRange "Current Range (A):"; Td "Time Delay (s):"; Top "Pickup Current (A):"; ResCurr "Residual Current (A):"
  Trip : Outport  InitialOutput=0
  Logic : Outport  Port=2  InitialOutput=0
  FaultType : Outport  Port=3  InitialOutput=0
  wires:
  Iabc/1 -> Overcurrent Relay Scheme/1(Iabc)
  Overcurrent Relay Scheme/1("TRIP ") -> Trip/1
  Overcurrent Relay Scheme/2(Logic) -> Logic/1
  Overcurrent Relay Scheme/3(FaultType) -> FaultType/1

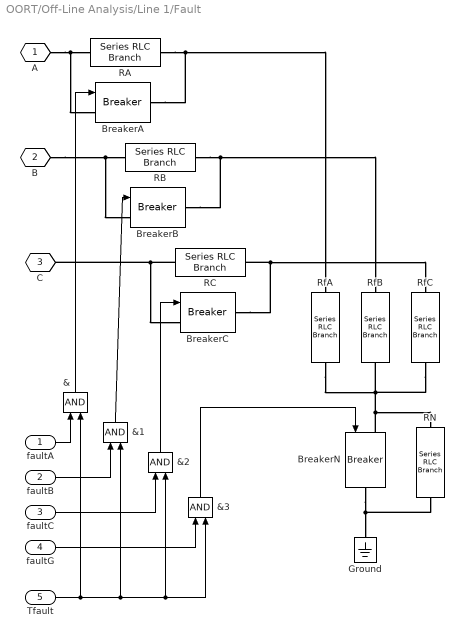
== system OORT/Off-Line Analysis/Line 1/Fault ==
  faultA : Inport
  faultB : Inport  Port=2
  faultC : Inport  Port=3
  faultG : Inport  Port=4
  Tfault : Inport  Port=5
  &{,1..3} (4 alike) : Logic
  BreakerA : powerlib/Elements/Breaker  DialogController=POWERSYS.PowerSysDialog  SystemSampleTime=-1  BreakerResistance=0.01  InitialState=0  SnubberResistance=1e6  SnubberCapacitance=inf  SwitchingTimes="[ 1/60  5/60 ]"  External=on  Measurements=None  MoreParameters=off  NoBreakLoop=off
  BreakerB : powerlib/Elements/Breaker  DialogController=POWERSYS.PowerSysDialog  SystemSampleTime=-1  BreakerResistance=0.01  InitialState=0  SnubberResistance=1e6  SnubberCapacitance=inf  SwitchingTimes="[ 1/60  5/60 ]"  External=on  Measurements=None  MoreParameters=off  NoBreakLoop=off
  BreakerC : powerlib/Elements/Breaker  DialogController=POWERSYS.PowerSysDialog  SystemSampleTime=-1  BreakerResistance=0.01  InitialState=0  SnubberResistance=1e6  SnubberCapacitance=inf  SwitchingTimes="[ 1/60  5/60 ]"  External=on  Measurements=None  MoreParameters=off  NoBreakLoop=off
  BreakerN : powerlib/Elements/Breaker  DialogController=POWERSYS.PowerSysDialog  SystemSampleTime=-1  BreakerResistance=0.01  InitialState=0  SnubberResistance=1e6  SnubberCapacitance=inf  SwitchingTimes="[ 1/60  5/60 ]"  External=on  Measurements=None  MoreParameters=off  NoBreakLoop=off
  Ground : powerlib/Elements/Ground  DialogController=POWERSYS.PowerSysDialog  PhysicalDomain=powersysdomain  SubClassName=unknown  LeftPortType=p1  RightPortType=p1  LConnTagsString=a
  RA : powerlib/Elements/Series RLC Branch  DialogController=POWERSYS.PowerSysDialog  PhysicalDomain=powersysdomain  SubClassName=unknown  LeftPortType=p1  RightPortType=p1  LConnTagsString=__new0  RConnTagsString=__new0  BranchType=R  Resistance=10000  Inductance=1e-3  SetiL0=off  InitialCurrent=0  Capacitance=1e-6  Setx0=off  InitialVoltage=0  Measurements=None
  RB : powerlib/Elements/Series RLC Branch  DialogController=POWERSYS.PowerSysDialog  PhysicalDomain=powersysdomain  SubClassName=unknown  LeftPortType=p1  RightPortType=p1  LConnTagsString=__new0  RConnTagsString=__new0  BranchType=R  Resistance=10000  Inductance=1e-3  SetiL0=off  InitialCurrent=0  Capacitance=1e-6  Setx0=off  InitialVoltage=0  Measurements=None
  RC : powerlib/Elements/Series RLC Branch  DialogController=POWERSYS.PowerSysDialog  PhysicalDomain=powersysdomain  SubClassName=unknown  LeftPortType=p1  RightPortType=p1  LConnTagsString=__new0  RConnTagsString=__new0  BranchType=R  Resistance=10000  Inductance=1e-3  SetiL0=off  InitialCurrent=0  Capacitance=1e-6  Setx0=off  InitialVoltage=0  Measurements=None
  RN : powerlib/Elements/Series RLC Branch  DialogController=POWERSYS.PowerSysDialog  PhysicalDomain=powersysdomain  SubClassName=unknown  LeftPortType=p1  RightPortType=p1  LConnTagsString=__new0  RConnTagsString=__new0  BranchType=R  Resistance=10000  Inductance=1e-3  SetiL0=off  InitialCurrent=0  Capacitance=1e-6  Setx0=off  InitialVoltage=0  Measurements=None
  RfA : powerlib/Elements/Series RLC Branch  DialogController=POWERSYS.PowerSysDialog  PhysicalDomain=powersysdomain  SubClassName=unknown  LeftPortType=p1  RightPortType=p1  LConnTagsString=__new0  RConnTagsString=__new0  BranchType=R  Resistance=faultR  Inductance=1e-3  SetiL0=off  InitialCurrent=0  Capacitance=1e-6  Setx0=off  InitialVoltage=0  Measurements=None
  RfB : powerlib/Elements/Series RLC Branch  DialogController=POWERSYS.PowerSysDialog  PhysicalDomain=powersysdomain  SubClassName=unknown  LeftPortType=p1  RightPortType=p1  LConnTagsString=__new0  RConnTagsString=__new0  BranchType=R  Resistance=faultR  Inductance=1e-3  SetiL0=off  InitialCurrent=0  Capacitance=1e-6  Setx0=off  InitialVoltage=0  Measurements=None
  RfC : powerlib/Elements/Series RLC Branch  DialogController=POWERSYS.PowerSysDialog  PhysicalDomain=powersysdomain  SubClassName=unknown  LeftPortType=p1  RightPortType=p1  LConnTagsString=__new0  RConnTagsString=__new0  BranchType=R  Resistance=faultR  Inductance=1e-3  SetiL0=off  InitialCurrent=0  Capacitance=1e-6  Setx0=off  InitialVoltage=0  Measurements=None
  A : PMIOPort  Tag=PMCPort  Port=1  Side=Left
  B : PMIOPort  Tag=PMCPort  Port=2  Side=Left
  C : PMIOPort  Tag=PMCPort  Port=3  Side=Left
  wires:
  faultA/1 -> &/1
  faultB/1 -> &1/1
  faultC/1 -> &2/1
  faultG/1 -> &3/1
  Tfault/1 -> &3/2, &2/2, &1/2, &/2
  &3/1 -> BreakerN/1
  &/1 -> BreakerA/1
  &1/1 -> BreakerB/1
  &2/1 -> BreakerC/1
  connections:
  B/RConn1 -- RB/LConn1 -- BreakerB/LConn1
  A/RConn1 -- BreakerA/LConn1 -- RA/LConn1
  RC/LConn1 -- C/RConn1 -- BreakerC/LConn1
  BreakerC/RConn1 -- RC/RConn1 -- RfC/LConn1
  RB/RConn1 -- RfB/LConn1 -- BreakerB/RConn1
  RA/RConn1 -- RfA/LConn1 -- BreakerA/RConn1
  BreakerN/LConn1 -- RN/LConn1 -- RfB/RConn1 -- RfA/RConn1 -- RfC/RConn1
  BreakerN/RConn1 -- Ground/LConn1 -- RN/RConn1

== system OORT/Off-Line Analysis/Line 1/Fault Selector ==
  "  " : Constant  Value=faultType
  "  +" : Logic  Operator=OR  Inputs=7
  " +" : Logic  Operator=OR  Inputs=5
  + : Logic  Operator=OR  Inputs=5
  "+ " : Logic  Operator=OR  Inputs=6
  A-B-C : Fcn  Expr=(u(1)==8)
  A-B-C-G : Fcn  Expr=(u(1)==9)
  A-G : Fcn  Expr=(u(1)==1)
  B-C : Fcn  Expr=(u(1)==4)
  B-C-G : Fcn  Expr=(u(1)==5)
  B-G : Fcn  Expr=(u(1)==2)
  C-A : Fcn  Expr=(u(1)==6)
  C-A-G : Fcn  Expr=(u(1)==7)
  C-G : Fcn  Expr=(u(1)==3)
  faultA : Outport  InitialOutput=0
  faultB : Outport  Port=2  InitialOutput=0
  faultC : Outport  Port=3  InitialOutput=0
  faultG : Outport  Port=4  InitialOutput=0
  wires:
  "  "/1 -> C-G/1, A-G/1, B-G/1, B-C/1, C-A/1, C-A-G/1, A-B-C/1, A-B-C-G/1, B-C-G/1
  +/1 -> faultA/1
  " +"/1 -> faultB/1
  "  +"/1 -> faultC/1
  "+ "/1 -> faultG/1
  A-G/1 -> "+ "/1, +/1
  C-A/1 -> "  +"/4, +/2
  B-G/1 -> " +"/1, "+ "/2
  B-C/1 -> "  +"/2, " +"/2
  B-C-G/1 -> "  +"/3, "+ "/4, " +"/3
  C-G/1 -> "  +"/1, "+ "/3
  C-A-G/1 -> "  +"/5, "+ "/5, +/3
  A-B-C-G/1 -> " +"/5, "  +"/7, "+ "/6, +/5
  A-B-C/1 -> " +"/4, "  +"/6, +/4
